simulink model "park_phasor"  (R2017a)
settings: Solver=ode23s  StartTime=0.0  StopTime=1.0  MaxStep=0.0001  RelTol=1e-8
values from neighbouring files (symbols this model uses):
  F_b = 50.0    (= 50)    [pll_phasor.m]
  K_p = 1.0/(tau_d*Omega_b)    (= 0.159154943092)    [pll_phasor.m]
  Omega_b = 2*pi*50    (= 314.159265359)    [pll_phasor.m]
  params = [K_p,Omega_b]    [pll_phasor.m]
libraries: powerlib_meascontrol x2
settings Model: Creator=jmmauricio  LastModifiedBy=jmmauricio

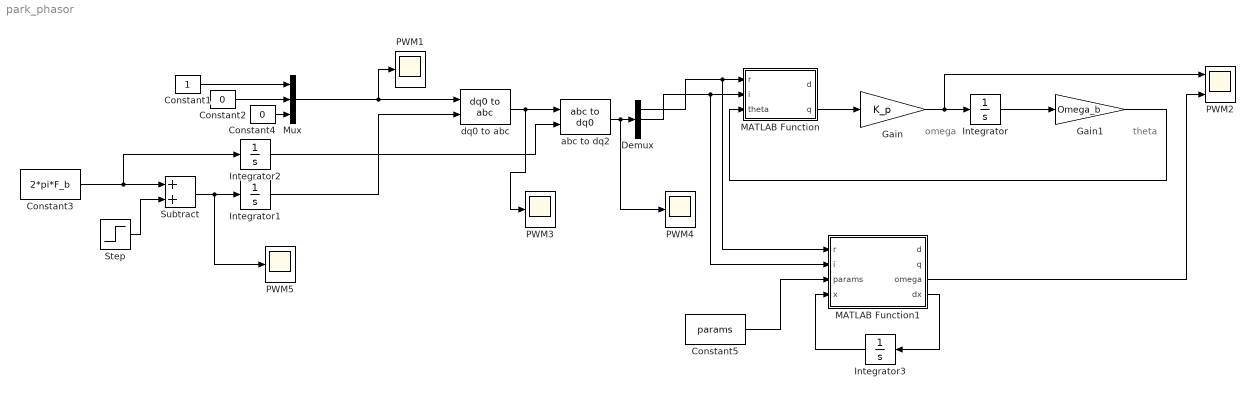
== system park_phasor ==
  note: omega
  note: theta
  Constant1 : Constant
  Constant2 : Constant  Value=0
  Constant3 : Constant  Value=2*pi*F_b
  Constant4 : Constant  Value=0
  Constant5 : Constant  Value=params
  Demux : Demux  Outputs=3
  Gain : Gain  Gain=K_p
  Gain1 : Gain  Gain=Omega_b
  Integrator : Integrator
  Integrator1 : Integrator
  Integrator2 : Integrator
  Integrator3 : Integrator  InitialCondition=[0]
  MATLAB Function : MATLAB Function  TreatAsAtomicUnit=on
  MATLAB Function1 : MATLAB Function  TreatAsAtomicUnit=on
  Mux : Mux  Inputs=3
  PWM{1,3..5} (4 alike) : Scope
  PWM2 : Scope  NumInputPorts=2
  Step : Step  Time=0.2  After=2*pi*(F_b)*0.05  SampleTime=0
  Subtract : Sum
  abc to dq2 : powerlib_meascontrol/Transformations/abc to dq0  Alignment=Aligned with phase A axis
  dq0 to abc : powerlib_meascontrol/Transformations/dq0 to abc  Alignment=Aligned with phase A axis
  wires:
  MATLAB Function/2(q) -> Gain/1
  Gain/1 -> PWM2/1, Integrator/1
  Integrator/1 -> Gain1/1
  Gain1/1 -> MATLAB Function/3(theta)
  dq0 to abc/1 -> PWM3/1, abc to dq2/1
  Mux/1 -> PWM1/1, dq0 to abc/1
  Constant4/1 -> Mux/3
  Constant1/1 -> Mux/1
  Integrator1/1 -> dq0 to abc/2
  Constant2/1 -> Mux/2
  Subtract/1 -> PWM5/1, Integrator1/1
  Constant3/1 -> Integrator2/1, Subtract/1
  Step/1 -> Subtract/2
  Integrator2/1 -> abc to dq2/2
  abc to dq2/1 -> PWM4/1, Demux/1
  Demux/1 -> MATLAB Function1/1(r), MATLAB Function/1(r)
  Demux/2 -> MATLAB Function1/2(i), MATLAB Function/2(i)
  Integrator3/1 -> MATLAB Function1/4(x)
  MATLAB Function1/4(dx) -> Integrator3/1
  Constant5/1 -> MATLAB Function1/3(params)
  MATLAB Function1/3(omega) -> PWM2/2

== matlab function park_phasor/MATLAB Function1 ==
  data: r input; d output; i input; q output; omega output; params input; x input; dx output
function [d,q,omega,dx] = fcn(r,i,params,x)

K_p = params(1);
Omega_b = params(2);

theta = x(1);

d = cos(theta)*r + cos(theta-pi/2)*i;
q =-sin(theta)*r - sin(theta-pi/2)*i;

omega = K_p*q;

dtheta = Omega_b*omega;

dx = [dtheta];

== matlab function park_phasor/MATLAB Function ==
  data: r input; d output; i input; q output; theta input
function [d,q] = fcn(r,i,theta)

d = cos(theta)*r + cos(theta-pi/2)*i;
q =-sin(theta)*r - sin(theta-pi/2)*i;
